simulink model "SDOF_SMD_input"  (R2016a)
settings: Solver=FixedStepAuto  StartTime=0.0  StopTime=10.0  FixedStep=.01  RelTol=1e-3
undefined symbols (not defined in the file): C, K, M
settings Model: Creator=ROB  LastModifiedBy=ROB

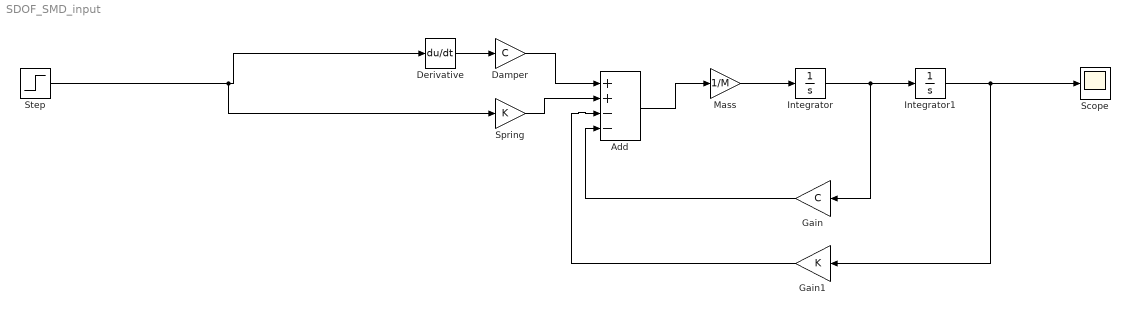
== system SDOF_SMD_input ==
  Add : Sum  Inputs=++--
  Damper : Gain  Gain=C
  Derivative : Derivative
  Gain : Gain  Gain=C
  Gain1 : Gain  Gain=K
  Integrator : Integrator
  Integrator1 : Integrator
  Mass : Gain  Gain=1/M
  Scope : Scope
  "Spring " : Gain  Gain=K
  Step : Step  SampleTime=0
  wires:
  Add/1 -> Mass/1
  Mass/1 -> Integrator/1
  Integrator/1 -> Gain/1, Integrator1/1
  Gain/1 -> Add/4
  Integrator1/1 -> Gain1/1, Scope/1
  Gain1/1 -> Add/3
  "Spring "/1 -> Add/2
  Derivative/1 -> Damper/1
  Damper/1 -> Add/1
  Step/1 -> "Spring "/1, Derivative/1
